simulink model "SAD_PROJECT"  (R2023b)
settings: Solver=ode5  StartTime=0.0  StopTime=5920  FixedStep=0.01  RelTol=1e-10  AbsTol=1e-11
values from neighbouring files (symbols this model uses):
  A = [0,  (1-K_yaw)*n, 0, -K_yaw*n^2,  0,   0 ... (first row only)    [SAD_CALLER.m]
  A_0 = A_B_LVLH*A_LVLH_ECI_0    [SAD_CALLER.m]    (also in veriAxilsym.m = eye(3))
  A_slew_B_LVLH = rot_matrix(deg2rad(-15.3),1)*rot_matrix(deg2rad(0),2)*rot_matrix(deg2rad(0),3)*eye(3)    [SAD_CALLER.m]
  alpha_mount_hs = 0.15    [SAD_CALLER.m]
  alpha_mount_ss = -0.5    [SAD_CALLER.m]
  B = [1/I(1,1),0,0 ... (first row only)    [SAD_CALLER.m]
  C = [0,0,0,1,0,0 ... (first row only)    [SAD_CALLER.m]
  correct_g = [5.7   7.4   0      0     0 ... (first row only)    [SAD_CALLER.m]    (also in veriAxilsym.m)
  correct_h = [  0  -25.9     0       0      0 ... (first row only)    [SAD_CALLER.m]    (also in veriAxilsym.m)
  d_cm_rw = 0.00000005    (= 5e-08)    [SAD_CALLER.m]
  d_cmsc_rw = 0.003    [SAD_CALLER.m]
  f = @(F) -F+e*sinh(F)+F_s-e*sinh(F_s)-M_h    [SAD_CALLER.m]
  FOV = 34    [SAD_CALLER.m]
  g_nm = [-29404.8 -1450.9     0      0     0 ... (first row only)    [SAD_CALLER.m]    (also in veriAxilsym.m)
  h_nm = [  0  4652.5      0      0       0 ... (first row only)    [SAD_CALLER.m]    (also in veriAxilsym.m)
  I = I_a+diag([0,4*M_a*x_cm^2,4*M_a*x_cm^2])+I_c+diag([0,M_c*d_cc_cm^2,M_c*d_cc_cm^2])+I_p+diag([0,6*M_p*(d_cc+d_cc_cm)^2,6*M_p*(d_cc-d_cc_cm)^2])    [SAD_CALLER.m]    (also in veriAxilsym.m = diag(I))
  I_r = 9.55e-5    (= 9.55e-05)    [SAD_CALLER.m]
  Inv_I = inv(I)    [SAD_CALLER.m]    (also in veriAxilsym.m = pinv(I))
  inv_R = inv(R)    [SAD_CALLER.m]
  J2 = 1.082626925638815e-3    (= 0.00108262692564)    [SAD_CALLER.m]    (also in veriAxilsym.m)
  K = [ -0.4323    0.0000   -0.0000   -0.0105    0.0000   -0.0000 ... (first row only)    [SAD_CALLER.m]
  L = [  0.0663    0.0001    0.0068 ... (first row only)    [SAD_CALLER.m]
  M_brake = 0.0002    [SAD_CALLER.m]
  M_rw = 0.2    [SAD_CALLER.m]    (also in veriAxilsym.m)
  m_sc_body = [1;1;1]*10e-3*M_tot/sqrt(3)    [SAD_CALLER.m]    (also in veriAxilsym.m)
  maneuver = input('type of maneuver, 1 for nadir pointing, 2 for de-tumbling, 3 for slew ')    [SAD_CALLER.m]
  mu_E = 3.986004418e5    (= 398600.4418)    [SAD_CALLER.m]    (also in veriAxilsym.m = 398600)
  mu_S = 1.327124400e11    (= 132712440000)    [SAD_CALLER.m]
  n = 2*pi/T    [SAD_CALLER.m]
  om_rw_0 = [0,0,0]    [SAD_CALLER.m]
  omega_E = 2*pi/(24*60*60)    (= 7.27220521664e-05)    [SAD_CALLER.m]    (also in veriAxilsym.m)
  omega_sc_0 = [0,0,n]    [SAD_CALLER.m]    (also in veriAxilsym.m = [0; 0; 0])
  pinv_R_xy = pinv(R_xy)    [SAD_CALLER.m]
  pinv_R_xz = pinv(R_xz)    [SAD_CALLER.m]
  pinv_R_yz = pinv(R_yz)    [SAD_CALLER.m]
  R = [cos(angle),-sin(angle),0;sin(angle),cos(angle),0;0,0,1]    [SAD_CALLER.m]    (also in veriAxilsym.m = 6378.1363)
  R_E_eqtr = 6378.1363    [SAD_CALLER.m]    (also in veriAxilsym.m)
  R_x = R(:,1)    [SAD_CALLER.m]
  R_y = R(:,2)    [SAD_CALLER.m]
  R_z = R(:,3)    [SAD_CALLER.m]
  rr_Esc_0 = s(end,(1:3))'    [SAD_CALLER.m]    (also in veriAxilsym.m = [7070.6; 0; 0])
  RR_x = [R_x,R_rad_x_1',R_rad_x_2']    [SAD_CALLER.m]
  RR_y = [R_y,R_rad_y_1',R_rad_y_2']    [SAD_CALLER.m]
  RR_z = [R_z,R_rad_z_1',R_rad_z_2']    [SAD_CALLER.m]
  smith_norm = zeros(4,5)    [SAD_CALLER.m]    (also in veriAxilsym.m)
  theta_G0 = mod(theta_G_Winter_solstice+omega_E*t_elapsed,2*pi)    [SAD_CALLER.m]    (also in veriAxilsym.m)
  vv_Esc_0 = s(end,(4:6))'    [SAD_CALLER.m]    (also in veriAxilsym.m = [0; 7.4338; 0])
undefined symbols (not defined in the file or in its folder): omega_0, rr_ES_0, vv_ES_0
libraries: matrix_library x24, simulink_extras x9, simulink x5
(part 2 of 2)

== system SAD_PROJECT/REACTION WHEELS/Subsystem1/static unbalance rw1 ==
  om_rw_1 : Inport
  Constant : Constant  Value=0
  Constant1 : Constant  Value=M_rw
  Constant2 : Constant  Value=RR_x
  Constant3 : Constant  Value=2*pi
  Constant4 : Constant  Value=[d_cmsc_rw;0;0]
  Constant6 : Constant  Value=[1;0;0]
  Constant7 : Constant  Value=0
  Cos : Trigonometry  Operator=cos
  Cross Product : matrix_library/Cross Product
  Cross Product1 : matrix_library/Cross Product
  Cross Product2 : matrix_library/Cross Product
  Gain : Gain  Gain=d_cm_rw
  Integrator : Integrator  InitialConditionSource=external
  Matrix Multiply : Product  Multiplication=Matrix(*)
  Matrix Multiply1 : Product
  Matrix Multiply2 : Product  Multiplication=Matrix(*)
  Mod : Math  Operator=mod
  Mux : Mux  Inputs=3
  Sin : Trigonometry
  Sum : Sum
  Output : Outport
  wires:
  Constant7/1 -> Mux/1
  Sin/1 -> Mux/3
  Cos/1 -> Mux/2
  Sum/1 -> Cross Product2/1
  Constant4/1 -> Sum/1
  Cross Product2/1 -> Output/1
  Matrix Multiply2/1 -> Cross Product2/2
  Mux/1 -> Gain/1
  Gain/1 -> Sum/2, Cross Product/2
  Mod/1 -> Cos/1, Sin/1
  Constant1/1 -> Matrix Multiply1/1
  Cross Product1/1 -> Matrix Multiply1/2
  Cross Product/1 -> Cross Product1/2
  Matrix Multiply1/1 -> Matrix Multiply2/2  "Radial force RW system"
  om_rw_1/1 -> Matrix Multiply/2, Integrator/1
  Constant3/1 -> Mod/2
  Constant/1 -> Integrator/2
  Integrator/1 -> Mod/1
  Constant6/1 -> Matrix Multiply/1
  Matrix Multiply/1 -> Cross Product/1, Cross Product1/1
  Constant2/1 -> Matrix Multiply2/1

== system SAD_PROJECT/REACTION WHEELS/Subsystem1/static unbalance rw2 ==
  om_rw_2 : Inport
  Constant : Constant  Value=0
  Constant1 : Constant  Value=M_rw
  Constant2 : Constant  Value=RR_y
  Constant3 : Constant  Value=2*pi
  Constant4 : Constant  Value=[0;d_cmsc_rw;0]
  Constant6 : Constant  Value=[1;0;0]
  Constant7 : Constant  Value=0
  Cos : Trigonometry  Operator=cos
  Cross Product : matrix_library/Cross Product
  Cross Product1 : matrix_library/Cross Product
  Cross Product2 : matrix_library/Cross Product
  Gain : Gain  Gain=d_cm_rw
  Integrator : Integrator  InitialConditionSource=external
  Matrix Multiply : Product  Multiplication=Matrix(*)
  Matrix Multiply1 : Product
  Matrix Multiply2 : Product  Multiplication=Matrix(*)
  Mod : Math  Operator=mod
  Mux : Mux  Inputs=3
  Sin : Trigonometry
  Sum : Sum
  Output : Outport
  wires:
  Constant6/1 -> Matrix Multiply/1
  Constant1/1 -> Matrix Multiply1/1
  Integrator/1 -> Mod/1
  Sin/1 -> Mux/3
  Constant4/1 -> Sum/1
  Mod/1 -> Cos/1, Sin/1
  Matrix Multiply2/1 -> Cross Product2/2
  Constant/1 -> Integrator/2
  Cross Product/1 -> Cross Product1/2
  Cross Product1/1 -> Matrix Multiply1/2
  Matrix Multiply1/1 -> Matrix Multiply2/2  "Radial force RW system"
  Cross Product2/1 -> Output/1
  Gain/1 -> Sum/2, Cross Product/2
  Constant3/1 -> Mod/2
  Mux/1 -> Gain/1
  Sum/1 -> Cross Product2/1
  Cos/1 -> Mux/2
  Constant2/1 -> Matrix Multiply2/1
  Constant7/1 -> Mux/1
  om_rw_2/1 -> Matrix Multiply/2, Integrator/1
  Matrix Multiply/1 -> Cross Product/1, Cross Product1/1

== system SAD_PROJECT/REACTION WHEELS/Subsystem1/static unbalance rw3 ==
  om_rw_1 : Inport
  Constant : Constant  Value=0
  Constant1 : Constant  Value=M_rw
  Constant2 : Constant  Value=RR_z
  Constant3 : Constant  Value=2*pi
  Constant4 : Constant  Value=[0;0;d_cmsc_rw]
  Constant6 : Constant  Value=[1;0;0]
  Constant7 : Constant  Value=0
  Cos : Trigonometry  Operator=cos
  Cross Product : matrix_library/Cross Product
  Cross Product1 : matrix_library/Cross Product
  Cross Product2 : matrix_library/Cross Product
  Gain : Gain  Gain=d_cm_rw
  Integrator : Integrator  InitialConditionSource=external
  Matrix Multiply : Product
  Matrix Multiply1 : Product
  Matrix Multiply2 : Product  Multiplication=Matrix(*)
  Mod : Math  Operator=mod
  Mux : Mux  Inputs=3
  Sin : Trigonometry
  Sum : Sum
  Output : Outport
  wires:
  Constant6/1 -> Matrix Multiply/1
  Constant1/1 -> Matrix Multiply1/1
  Integrator/1 -> Mod/1
  Sin/1 -> Mux/3
  Constant4/1 -> Sum/1
  Mod/1 -> Cos/1, Sin/1
  Matrix Multiply2/1 -> Cross Product2/2
  Constant/1 -> Integrator/2
  Cross Product/1 -> Cross Product1/2
  Cross Product1/1 -> Matrix Multiply1/2
  Matrix Multiply1/1 -> Matrix Multiply2/2  "Radial force RW system"
  Cross Product2/1 -> Output/1
  Gain/1 -> Cross Product/2, Sum/2
  Constant3/1 -> Mod/2
  Mux/1 -> Gain/1
  Sum/1 -> Cross Product2/1
  Cos/1 -> Mux/2
  Constant2/1 -> Matrix Multiply2/1
  Constant7/1 -> Mux/1
  om_rw_1/1 -> Matrix Multiply/2, Integrator/1
  Matrix Multiply/1 -> Cross Product/1, Cross Product1/1

== system SAD_PROJECT/SENSORS/Horizon Sensor/Inverse pinhole camera model ==
  In1 : Inport
  In2 : Inport  Port=2
  Atan : Trigonometry  Operator=atan
  Atan1 : Trigonometry  Operator=atan
  Constant8 : Constant  Value=FOV/2
  Constant9 : Constant  Value=f
  Divide4 : Product  Inputs=*/
  Divide5 : Product  Inputs=*/
  Sum6 : Sum  Inputs=|+-
  Sum7 : Sum  Inputs=-+|
  Out1 : Outport
  Out2 : Outport  Port=2
  wires:
  Constant9/1 -> Divide5/2, Divide4/2
  Sum7/1 -> Divide5/1
  In2/1 -> Sum7/2
  Sum6/1 -> Divide4/1
  Constant8/1 -> Sum7/1, Sum6/2
  Divide5/1 -> Atan1/1
  Divide4/1 -> Atan/1
  Atan/1 -> Out1/1
  In1/1 -> Sum6/1
  Atan1/1 -> Out2/1

== system SAD_PROJECT/SENSORS/Horizon Sensor/Pinhole camera model ==
  In1 : Inport
  In2 : Inport  Port=2
  Constant4 : Constant  Value=f
  Constant5 : Constant  Value=FOV/2
  Degrees to Radians : simulink_extras/Transformations/Degrees to Radians
  Degrees to Radians1 : simulink_extras/Transformations/Degrees to Radians
  Product2 : Product
  Product3 : Product
  Sum2 : Sum  Inputs=|++
  Sum3 : Sum  Inputs=++|
  Tan : Trigonometry  Operator=tan
  Tan1 : Trigonometry  Operator=tan
  Out1 : Outport
  Out2 : Outport  Port=2
  wires:
  Constant5/1 -> Sum3/1, Sum2/2
  Product2/1 -> Sum2/1
  Product3/1 -> Sum3/2
  Constant4/1 -> Product3/1, Product2/2
  Sum2/1 -> Out1/1
  Sum3/1 -> Out2/1
  Degrees to Radians/1 -> Tan/1
  In1/1 -> Degrees to Radians/1
  Degrees to Radians1/1 -> Tan1/1
  In2/1 -> Degrees to Radians1/1
  Tan/1 -> Product2/1
  Tan1/1 -> Product3/2

== system SAD_PROJECT/ENVIRONMENT/Magnetic Torque/Cartesian 2 spherical/Subsystem ==
  Clock : Clock
  Constant : Constant  Value=theta_G0
  Constant1 : Constant  Value=omega_E
  Constant2 : Constant  Value=2*pi
  Mod : Math  Operator=mod
  Product : Product
  Sum : Sum  Inputs=|++
  Output : Outport
  wires:
  Constant/1 -> Sum/1
  Product/1 -> Sum/2
  Clock/1 -> Product/2
  Sum/1 -> Mod/1  "theta_G(t)"
  Constant1/1 -> Product/1
  Constant2/1 -> Mod/2
  Mod/1 -> Output/1

== system SAD_PROJECT/ENVIRONMENT/Magnetic Torque/MAGNETIC TORQUE in BODY/B in ECI system ==
  local siderial time : Inport
  longitude : Inport  Port=2
  r : Inport  Port=3
  latitude : Inport  Port=4
  Bphi cos : Product
  Bphi sin : Product
  Br cos : Product
  Br sin : Product
  Btheta cos : Product
  Btheta sin : Product
  Product : Product
  Product1 : Product
  SinCos : Trigonometry  Operator=sincos
  SinCos1 : Trigonometry  Operator=sincos
  Sum : Sum  Inputs=|++
  Sum1 : Sum  Inputs=|-+
  Sum2 : Sum  Inputs=|++
  Sum3 : Sum  Inputs=|++
  spherical coordinates : Subsystem
  Out1 : Outport
  Out2 : Outport  Port=2
  Out3 : Outport  Port=3
  wires:
  Sum3/1 -> Out2/1
  Sum1/1 -> Out1/1
  Bphi sin/1 -> Sum1/1
  Btheta sin/1 -> Sum/2
  Sum2/1 -> Out3/1
  Product1/1 -> Sum3/2
  SinCos1/2 -> Btheta cos/2, Br cos/2
  r/1 -> spherical coordinates/2(r)
  latitude/1 -> SinCos1/1, spherical coordinates/3(latitude)
  spherical coordinates/1(B_r) -> Br cos/1, Br sin/1
  Br sin/1 -> Sum2/1
  longitude/1 -> spherical coordinates/1(longitude)
  local siderial time/1 -> SinCos/1
  spherical coordinates/2(B_t) -> Btheta sin/1, Btheta cos/1
  Sum/1 -> Product1/1, Product/1
  Br cos/1 -> Sum/1
  Btheta cos/1 -> Sum2/2
  SinCos1/1 -> Btheta sin/2, Br sin/2
  SinCos/2 -> Bphi cos/2, Product/2
  Bphi cos/1 -> Sum3/1
  SinCos/1 -> Bphi sin/2, Product1/2
  Product/1 -> Sum1/2
  spherical coordinates/3(B_p) -> Bphi sin/1, Bphi cos/1

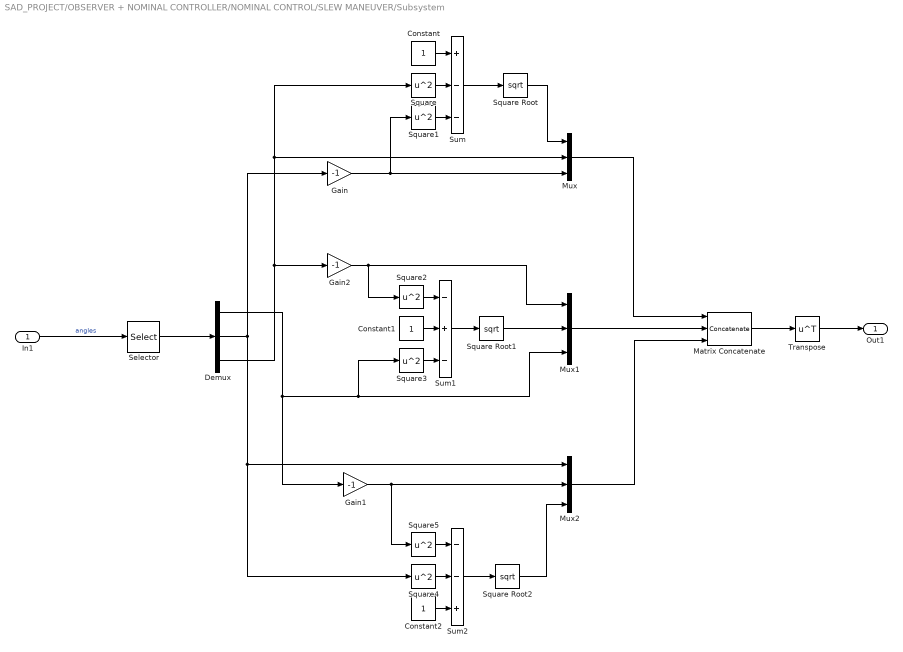
== system SAD_PROJECT/OBSERVER + NOMINAL CONTROLLER/NOMINAL CONTROL/SLEW MANEUVER/Subsystem ==
  In1 : Inport
  Constant : Constant
  Constant1 : Constant
  Constant2 : Constant
  Demux : Demux  Outputs=3
  Gain : Gain  Gain=-1
  Gain1 : Gain  Gain=-1
  Gain2 : Gain  Gain=-1
  Matrix Concatenate : Concatenate  NumInputs=3  Mode=Multidimensional array  ConcatenateDimension=2
  Mux : Mux  Inputs=3
  Mux1 : Mux  Inputs=3
  Mux2 : Mux  Inputs=3
  Selector : Selector  InputPortWidth=6  IndexOptions=Index vector (dialog)  Indices=[4 5 6]  OutputSizes=1
  Square{,1..5} (6 alike) : Math  Operator=square
  Square Root : Sqrt
  Square Root1 : Sqrt
  Square Root2 : Sqrt
  Sum : Sum  Inputs=+--
  Sum1 : Sum  Inputs=-+-
  Sum2 : Sum  Inputs=--+
  Transpose : Math  Operator=transpose
  Out1 : Outport
  wires:
  In1/1 -> Selector/1  "angles"
  Demux/3 -> Square/1, Mux/2, Gain2/1
  Gain/1 -> Square1/1, Mux/3
  Selector/1 -> Demux/1
  Gain1/1 -> Square5/1, Mux2/2
  Mux2/1 -> Matrix Concatenate/3
  Mux1/1 -> Matrix Concatenate/2
  Matrix Concatenate/1 -> Transpose/1
  Transpose/1 -> Out1/1
  Square/1 -> Sum/2
  Square1/1 -> Sum/3
  Constant/1 -> Sum/1
  Sum/1 -> Square Root/1
  Square Root/1 -> Mux/1
  Gain2/1 -> Mux1/1, Square2/1
  Square Root1/1 -> Mux1/2
  Square2/1 -> Sum1/1
  Square3/1 -> Sum1/3
  Sum1/1 -> Square Root1/1
  Constant1/1 -> Sum1/2
  Square Root2/1 -> Mux2/3
  Demux/1 -> Gain1/1, Square3/1, Mux1/3
  Square5/1 -> Sum2/1
  Demux/2 -> Square4/1, Mux2/1, Gain/1
  Sum2/1 -> Square Root2/1
  Square4/1 -> Sum2/2
  Constant2/1 -> Sum2/3
  Mux/1 -> Matrix Concatenate/1

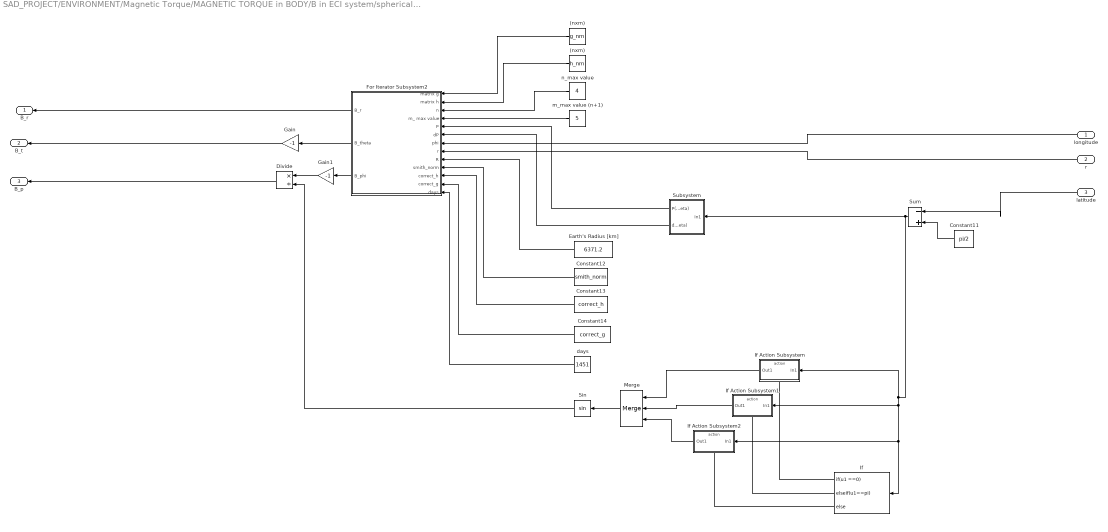
== system SAD_PROJECT/ENVIRONMENT/Magnetic Torque/MAGNETIC TORQUE in BODY/B in ECI system/spherical coordinates ==
  longitude : Inport
  r : Inport  Port=2
  latitude : Inport  Port=3
  " (nxm)" : Constant  Value=g_nm
  (nxm) : Constant  Value=h_nm
  Constant11 : Constant  Value=pi/2
  Constant12 : Constant  Value=smith_norm
  Constant13 : Constant  Value=correct_h
  Constant14 : Constant  Value=correct_g
  Divide : Product  Inputs=*/
  Earth's Radius [km] : Constant  Value=6371.2
  For Iterator Subsystem2 : Subsystem  TreatAsAtomicUnit=on
  Gain : Gain  Gain=-1
  Gain1 : Gain  Gain=-1
  If : If  IfExpression=u1 ==0  ElseIfExpressions=u1==pi
  If Action Subsystem : Subsystem  TreatAsAtomicUnit=on
  If Action Subsystem1 : Subsystem  TreatAsAtomicUnit=on
  If Action Subsystem2 : Subsystem  TreatAsAtomicUnit=on
  Merge : Merge  Inputs=3
  Sin : Trigonometry
  Subsystem : Subsystem
  Sum : Sum  Inputs=|-+
  days : Constant  Value=1451
  m_max value (n+1) : Constant  Value=5
  n_max value : Constant  Value=4  OutDataTypeStr=int32
  B_r : Outport
  B_t : Outport  Port=2
  B_p : Outport  Port=3
  wires:
  Divide/1 -> B_p/1
  Constant11/1 -> Sum/2
  Gain/1 -> B_t/1
  Subsystem/1(P(theta)) -> For Iterator Subsystem2/5(P)
  days/1 -> For Iterator Subsystem2/13(days)
  For Iterator Subsystem2/1(B_r) -> B_r/1
  n_max value/1 -> For Iterator Subsystem2/3(n)
  For Iterator Subsystem2/2(B_theta) -> Gain/1
  Constant13/1 -> For Iterator Subsystem2/11("correct_h ")
  Constant14/1 -> For Iterator Subsystem2/12(correct_g)
  r/1 -> For Iterator Subsystem2/8(r)
  longitude/1 -> For Iterator Subsystem2/7(phi)
  Subsystem/2(dP(theta)) -> For Iterator Subsystem2/6(dP)
  latitude/1 -> Sum/1
  Sin/1 -> Divide/2
  Constant12/1 -> For Iterator Subsystem2/10(smith_norm)
  Earth's Radius [km]/1 -> For Iterator Subsystem2/9(R)
  Gain1/1 -> Divide/1
  For Iterator Subsystem2/3(B_phi) -> Gain1/1
  m_max value (n+1)/1 -> For Iterator Subsystem2/4(m_ max value)
  " (nxm)"/1 -> For Iterator Subsystem2/1(matrix g)
  (nxm)/1 -> For Iterator Subsystem2/2(matrix h)
  If Action Subsystem1/1(Out1) -> Merge/2
  If Action Subsystem2/1(Out1) -> Merge/3
  If Action Subsystem/1(Out1) -> Merge/1
  Sum/1 -> If Action Subsystem/1(In1), If Action Subsystem2/1(In1), If/1, If Action Subsystem1/1(In1), Subsystem/1(In1)
  Merge/1 -> Sin/1
  If/3 -> If Action Subsystem2/Action
  If/1 -> If Action Subsystem/Action
  If/2 -> If Action Subsystem1/Action

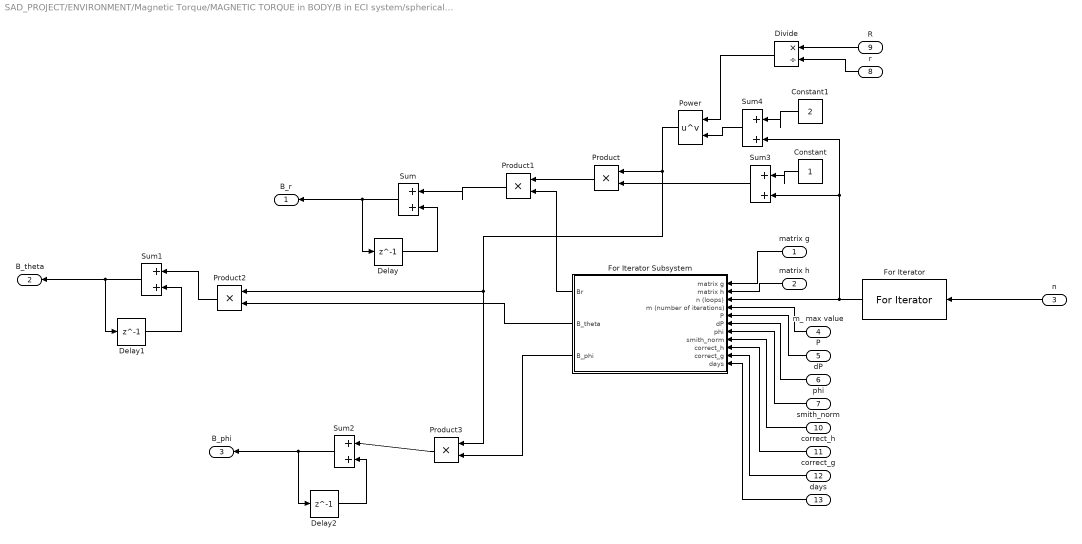
== system SAD_PROJECT/ENVIRONMENT/Magnetic Torque/MAGNETIC TORQUE in BODY/B in ECI system/spherical coordinates/For Iterator Subsystem2 ==
  matrix g : Inport
  matrix h : Inport  Port=2
  n : Inport  Port=3
  m_ max value : Inport  Port=4
  P : Inport  Port=5
  dP : Inport  Port=6
  phi : Inport  Port=7
  r : Inport  Port=8
  R : Inport  Port=9
  smith_norm : Inport  Port=10
  "correct_h " : Inport  Port=11
  correct_g : Inport  Port=12
  days : Inport  Port=13
  Constant : Constant
  Constant1 : Constant  Value=2
  Delay : Delay  DelayLength=1  InitialCondition=0
  Delay1 : Delay  DelayLength=1  InitialCondition=0
  Delay2 : Delay  DelayLength=1  InitialCondition=0
  Divide : Product  Inputs=*/
  For Iterator : ForIterator  ResetStates=reset  IterationSource=external
  For Iterator Subsystem : Subsystem  TreatAsAtomicUnit=on
  Power : Math  Operator=pow  OutputSignalType=real
  Product{,1..3} (4 alike) : Product
  Sum : Sum  Inputs=|++
  Sum1 : Sum  Inputs=|++
  Sum2 : Sum  Inputs=|++
  Sum3 : Sum  Inputs=|++  OutDataTypeStr=double
  Sum4 : Sum  Inputs=|++  OutDataTypeStr=double
  B_r : Outport
  B_theta : Outport  Port=2
  B_phi : Outport  Port=3
  wires:
  n/1 -> For Iterator/1
  Sum/1 -> Delay/1, B_r/1
  Delay/1 -> Sum/2
  matrix h/1 -> For Iterator Subsystem/2(matrix h)
  matrix g/1 -> For Iterator Subsystem/1(matrix g)
  For Iterator/1 -> Sum4/2, Sum3/2, For Iterator Subsystem/3(n (loops))
  m_ max value/1 -> For Iterator Subsystem/4(m (number of iterations))
  P/1 -> For Iterator Subsystem/5(P)
  dP/1 -> For Iterator Subsystem/6(dP)
  Sum1/1 -> Delay1/1, B_theta/1
  Delay1/1 -> Sum1/2
  Sum2/1 -> Delay2/1, B_phi/1
  Delay2/1 -> Sum2/2
  phi/1 -> For Iterator Subsystem/7(phi)
  Constant/1 -> Sum3/1
  R/1 -> Divide/1
  r/1 -> Divide/2
  Sum3/1 -> Product/2
  Divide/1 -> Power/1
  Power/1 -> Product/1, Product3/1, Product2/1
  Product/1 -> Product1/1
  For Iterator Subsystem/1(Br) -> Product1/2
  Product1/1 -> Sum/1
  Constant1/1 -> Sum4/1
  Sum4/1 -> Power/2
  smith_norm/1 -> For Iterator Subsystem/8(smith_norm)
  "correct_h "/1 -> For Iterator Subsystem/9("correct_h ")
  correct_g/1 -> For Iterator Subsystem/10(correct_g)
  days/1 -> For Iterator Subsystem/11(days)
  Product2/1 -> Sum1/1
  For Iterator Subsystem/2(B_theta) -> Product2/2
  Product3/1 -> Sum2/1
  For Iterator Subsystem/3(B_phi) -> Product3/2

== system SAD_PROJECT/ENVIRONMENT/Magnetic Torque/MAGNETIC TORQUE in BODY/B in ECI system/spherical coordinates/If Action Subsystem ==
  In1 : Inport
  Action Port : ActionPort  ActionPortLabel=if(u1 ==0)
  Constant : Constant  Value=0.0000001
  Sum : Sum  Inputs=|++
  Out1 : Outport
  wires:
  In1/1 -> Sum/1
  Sum/1 -> Out1/1
  Constant/1 -> Sum/2

== system SAD_PROJECT/ENVIRONMENT/Magnetic Torque/MAGNETIC TORQUE in BODY/B in ECI system/spherical coordinates/If Action Subsystem1 ==
  In1 : Inport
  Action Port : ActionPort  ActionPortLabel=elseif(u1==pi)
  Constant : Constant  Value=0.0000001
  Sum : Sum  Inputs=|++
  Out1 : Outport
  wires:
  In1/1 -> Sum/1
  Sum/1 -> Out1/1
  Constant/1 -> Sum/2

== system SAD_PROJECT/ENVIRONMENT/Magnetic Torque/MAGNETIC TORQUE in BODY/B in ECI system/spherical coordinates/If Action Subsystem2 ==
  In1 : Inport
  Action Port : ActionPort  ActionPortLabel=else
  Out1 : Outport
  wires:
  In1/1 -> Out1/1

== system SAD_PROJECT/ENVIRONMENT/Magnetic Torque/MAGNETIC TORQUE in BODY/B in ECI system/spherical coordinates/Subsystem ==
  In1 : Inport
  If : If  IfExpression=u1 ==0  ElseIfExpressions=u1==pi
  If Action Subsystem : Subsystem  TreatAsAtomicUnit=on
  If Action Subsystem1 : Subsystem  TreatAsAtomicUnit=on
  If Action Subsystem2 : Subsystem  TreatAsAtomicUnit=on
  Merge : Merge  Inputs=3
  P(v) : MATLAB Function  TreatAsAtomicUnit=on
  dP(v) : MATLAB Function  TreatAsAtomicUnit=on
  P(theta) : Outport
  dP(theta) : Outport  Port=2
  wires:
  dP(v)/1(y) -> dP(theta)/1
  If/2 -> If Action Subsystem1/Action
  P(v)/1(y) -> P(theta)/1
  If/1 -> If Action Subsystem/Action
  If Action Subsystem1/1(Out1) -> Merge/2
  If Action Subsystem/1(Out1) -> Merge/1
  Merge/1 -> dP(v)/1(u), P(v)/1(u)
  If Action Subsystem2/1(Out1) -> Merge/3
  In1/1 -> If Action Subsystem/1(In1), If Action Subsystem2/1(In1), If/1, If Action Subsystem1/1(In1)
  If/3 -> If Action Subsystem2/Action

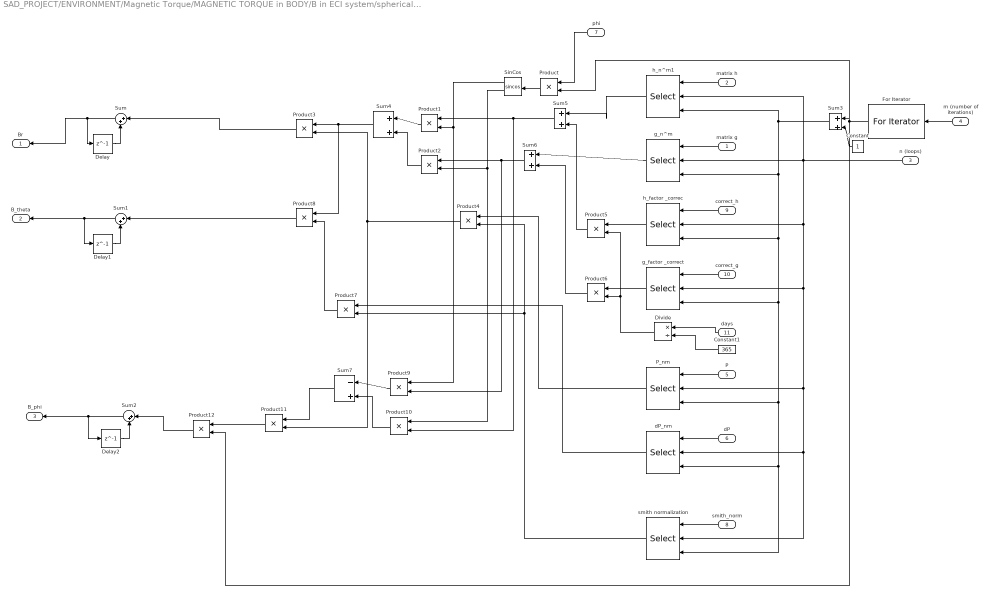
== system SAD_PROJECT/ENVIRONMENT/Magnetic Torque/MAGNETIC TORQUE in BODY/B in ECI system/spherical coordinates/For Iterator Subsystem2/For Iterator Subsystem ==
  matrix g : Inport
  matrix h : Inport  Port=2
  n (loops) : Inport  Port=3
  m (number of iterations) : Inport  Port=4
  P : Inport  Port=5
  dP : Inport  Port=6
  phi : Inport  Port=7
  smith_norm : Inport  Port=8
  "correct_h " : Inport  Port=9
  correct_g : Inport  Port=10
  days : Inport  Port=11
  Constant : Constant
  Constant1 : Constant  Value=365
  Delay : Delay  DelayLength=1  InitialCondition=0
  Delay1 : Delay  DelayLength=1  InitialCondition=0
  Delay2 : Delay  DelayLength=1  InitialCondition=0
  Divide : Product  Inputs=*/
  For Iterator : ForIterator  ResetStates=reset  IterationSource=external  IndexMode=Zero-based
  P_nm : Selector  NumberOfDimensions=2  InputPortWidth=6  IndexOptions=Starting index (port),Starting index (port)  Indices=[1 3],1  OutputSizes=1,1
  Product{,1..12} (13 alike) : Product
  SinCos : Trigonometry  Operator=sincos
  Sum{,1..6} (7 alike) : Sum  Inputs=|++
  Sum7 : Sum  Inputs=|-+
  dP_nm : Selector  NumberOfDimensions=2  InputPortWidth=6  IndexOptions=Starting index (port),Starting index (port)  Indices=[1 3],1  OutputSizes=1,1
  g_factor _correct : Selector  NumberOfDimensions=2  InputPortWidth=6  IndexOptions=Starting index (port),Starting index (port)  Indices=[1 3],1  OutputSizes=1,1
  g_n^m : Selector  NumberOfDimensions=2  InputPortWidth=6  IndexOptions=Starting index (port),Starting index (port)  Indices=[1 3],1  OutputSizes=1,1
  h_factor _correc : Selector  NumberOfDimensions=2  InputPortWidth=6  IndexOptions=Starting index (port),Starting index (port)  Indices=[1 3],1  OutputSizes=1,1
  h_n^m1 : Selector  NumberOfDimensions=2  InputPortWidth=6  IndexOptions=Starting index (port),Starting index (port)  Indices=[1 3],1  OutputSizes=1,1
  smith normalization : Selector  NumberOfDimensions=2  InputPortWidth=6  IndexOptions=Starting index (port),Starting index (port)  Indices=[1 3],1  OutputSizes=1,1
  Br : Outport
  B_theta : Outport  Port=2
  B_phi : Outport  Port=3
  wires:
  Sum/1 -> Br/1, Delay/1
  Delay/1 -> Sum/2
  m (number of iterations)/1 -> For Iterator/1
  matrix g/1 -> g_n^m/1
  matrix h/1 -> h_n^m1/1
  P/1 -> P_nm/1
  dP/1 -> dP_nm/1
  Sum1/1 -> B_theta/1, Delay1/1
  Delay1/1 -> Sum1/2
  Sum2/1 -> B_phi/1, Delay2/1
  Delay2/1 -> Sum2/2
  For Iterator/1 -> Product/2, Product12/2, Sum3/1
  Constant/1 -> Sum3/2
  phi/1 -> Product/1
  Product/1 -> SinCos/1
  Product1/1 -> Sum4/1
  Product2/1 -> Sum4/2
  Sum4/1 -> Product8/1, Product3/1
  P_nm/1 -> Product4/1
  Product3/1 -> Sum/1
  SinCos/2 -> Product2/2, Product10/1
  smith_norm/1 -> smith normalization/1
  Product4/1 -> Product3/2, Product11/2
  smith normalization/1 -> Product7/2, Product4/2
  "correct_h "/1 -> h_factor _correc/1
  n (loops)/1 -> h_factor _correc/2, smith normalization/2, dP_nm/2, P_nm/2, g_factor _correct/2, h_n^m1/2, g_n^m/2
  Sum3/1 -> g_n^m/3, h_factor _correc/3, g_factor _correct/3, smith normalization/3, dP_nm/3, P_nm/3, h_n^m1/3
  correct_g/1 -> g_factor _correct/1
  Constant1/1 -> Divide/2
  days/1 -> Divide/1
  g_factor _correct/1 -> Product6/1
  Divide/1 -> Product5/2, Product6/2
  h_factor _correc/1 -> Product5/1
  Sum5/1 -> Product1/1, Product10/2
  h_n^m1/1 -> Sum5/1
  Product5/1 -> Sum5/2
  Sum6/1 -> Product2/1, Product9/2
  g_n^m/1 -> Sum6/1
  Product6/1 -> Sum6/2
  dP_nm/1 -> Product7/1
  Product7/1 -> Product8/2
  Product8/1 -> Sum1/1
  SinCos/1 -> Product9/1, Product1/2
  Product10/1 -> Sum7/2
  Product9/1 -> Sum7/1
  Sum7/1 -> Product11/1
  Product11/1 -> Product12/1
  Product12/1 -> Sum2/1

== system SAD_PROJECT/ENVIRONMENT/Magnetic Torque/MAGNETIC TORQUE in BODY/B in ECI system/spherical coordinates/Subsystem/If Action Subsystem ==
  In1 : Inport
  Action Port : ActionPort  ActionPortLabel=if(u1 ==0)
  Constant : Constant  Value=0.0000001
  Sum : Sum  Inputs=|++
  Out1 : Outport
  wires:
  In1/1 -> Sum/1
  Sum/1 -> Out1/1
  Constant/1 -> Sum/2

== system SAD_PROJECT/ENVIRONMENT/Magnetic Torque/MAGNETIC TORQUE in BODY/B in ECI system/spherical coordinates/Subsystem/If Action Subsystem1 ==
  In1 : Inport
  Action Port : ActionPort  ActionPortLabel=elseif(u1==pi)
  Constant : Constant  Value=0.0000001
  Sum : Sum  Inputs=|++
  Out1 : Outport
  wires:
  In1/1 -> Sum/1
  Sum/1 -> Out1/1
  Constant/1 -> Sum/2

== system SAD_PROJECT/ENVIRONMENT/Magnetic Torque/MAGNETIC TORQUE in BODY/B in ECI system/spherical coordinates/Subsystem/If Action Subsystem2 ==
  In1 : Inport
  Action Port : ActionPort  ActionPortLabel=else
  Out1 : Outport
  wires:
  In1/1 -> Out1/1

== matlab function SAD_PROJECT/ENVIRONMENT/Magnetic Torque/MAGNETIC TORQUE in BODY/B in ECI system/spherical coordinates/Subsystem/P(v) ==
  data: u input; y output
function y = fcn(u)

P=@(v) [ cos(v)                         sin(v)                               0                             0                   0 
        (3*cos(v)^2-1)/2                3*cos(v)*sin(v)                      3*sin(v)^2                    0                   0
        (5*cos(v)^3-3*cos(v))/2         sin(v)*(15*cos(v)^2-3)/2             15*cos(v)*sin(v)^2            sin(v)^3*15         0
        (35*cos(v)^4-30*cos(v)^2+3)/8   sin(v)*(140*cos(v)^3-60*cos(v))/8    sin(v)^2*(420*cos(v)^2-60)/8  105*sin(v)^3*cos(v) 105*sin(v)^4  ];


y = P(u);

== matlab function SAD_PROJECT/ENVIRONMENT/Magnetic Torque/MAGNETIC TORQUE in BODY/B in ECI system/spherical coordinates/Subsystem/dP(v) ==
  data: u input; y output
function y = fcn(u)

dP=@(v) [-sin(v)                                cos(v)                                                          0                                                          0                                  0
         -3*sin(v)*cos(v)                       3*(cos(v)^2-sin(v)^2)                                           6*sin(v)*cos(v)                                            0                                  0
         (-15*cos(v)^2+3)/2*sin(v)              (15*cos(v)^2-3)/2*cos(v)-sin(v)^2*(15*cos(v))                   30*cos(v)^2*sin(v)-15*sin(v)^3                             45*cos(v)*sin(v)^2                 0
         -sin(v)*(140*cos(v)^3-60*cos(v))/8     cos(v)*(140*cos(v)^3-60*cos(v))/8-sin(v)^2*(420*cos(v)^2-60)/8  2*sin(v)*cos(v)*(420*cos(v)^2-60)/8-sin(v)^3*(105*cos(v))  105*(3*sin(v)^2*cos(v)^2-sin(v)^4) 420*sin(v)^3*cos(v)];

y = dP(u);
